simulink model "MyControl3"  (R2020b)
settings: Solver=FixedStepAuto  StartTime=0.0  StopTime=100  RelTol=1e-3
undefined symbols (not defined in the file or in its folder): ld, Ts
libraries: Solver_SF x1, simulink x1
settings Model: Creator=Namo  LastModifiedBy=Namo

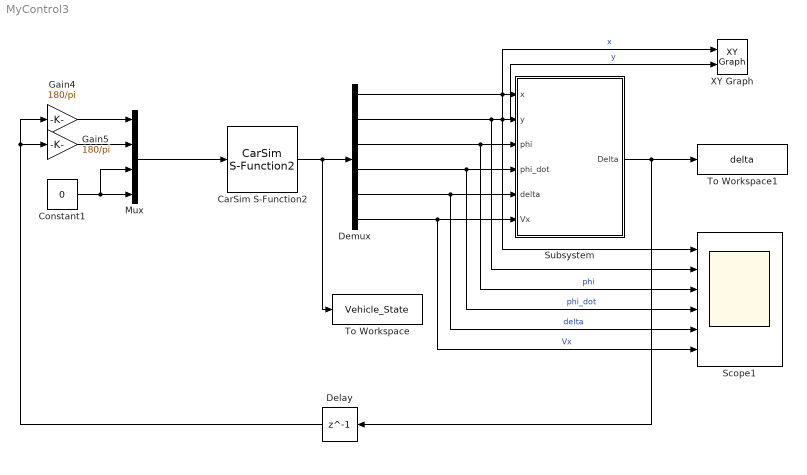
== system MyControl3 ==
  CarSim S-Function2 : Solver_SF/CarSim S-Function2  Priority=1  VehicleCode=i_i  SIMFILE=simfile.sim
      settings: AttributesFormatString=Vehicle Code: %<VehicleCode>
  Constant1 : Constant  Value=0
  Delay : Delay  DelayLength=1
  Demux : Demux  Outputs=6
  Gain4 : Gain  Gain=180/pi
  Gain5 : Gain  Gain=180/pi
  Mux : Mux
  Scope1 : Scope  NumInputPorts=6
  Subsystem : Subsystem
  To Workspace : ToWorkspace  VariableName=Vehicle_State  SampleTime=Ts
  To Workspace1 : ToWorkspace  VariableName=delta  SampleTime=-1
  XY Graph : simulink/Sinks/XY Graph  xmin=-5  xmax=200  ymin=-1  ymax=220  st=-1
  wires:
  Gain4/1 -> Mux/1
  Constant1/1 -> Mux/4, Mux/3
  CarSim S-Function2/1 -> To Workspace/1, Demux/1
  Subsystem/1(Delta) -> Delay/1, To Workspace1/1
  Mux/1 -> CarSim S-Function2/1
  Demux/6 -> Subsystem/6(Vx), Scope1/6  "Vx"
  Delay/1 -> Gain4/1, Gain5/1
  Demux/5 -> Scope1/5, Subsystem/5(delta)  "delta"
  Demux/3 -> Scope1/3, Subsystem/3(phi)  "phi"
  Gain5/1 -> Mux/2
  Demux/1 -> Scope1/1, XY Graph/1, Subsystem/1(x)  "x"
  Demux/2 -> XY Graph/2, Subsystem/2(y), Scope1/2  "y"
  Demux/4 -> Scope1/4, Subsystem/4(phi_dot)  "phi_dot"

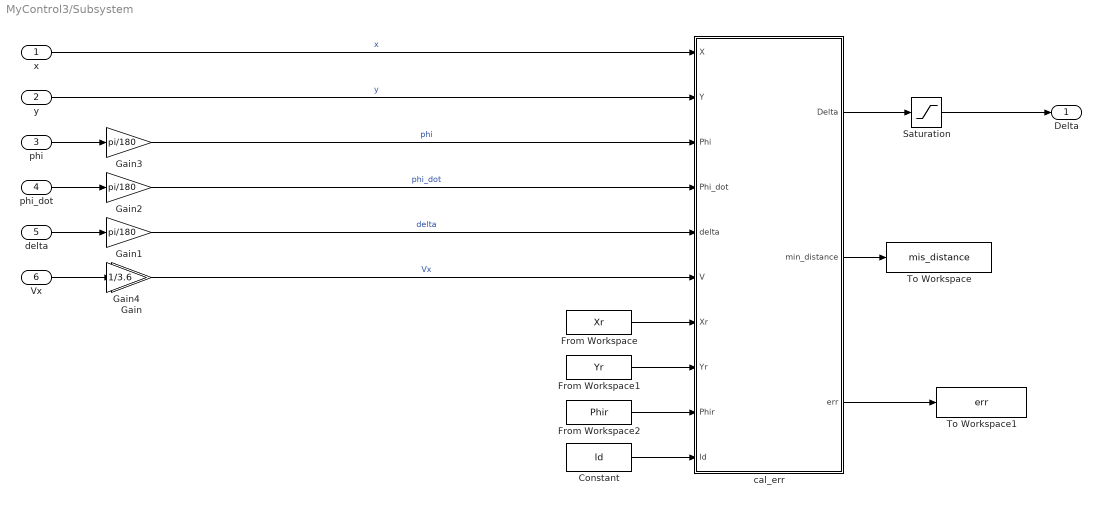
== system MyControl3/Subsystem ==
  x : Inport
  y : Inport  Port=2
  phi : Inport  Port=3
  phi_dot : Inport  Port=4
  delta : Inport  Port=5
  Vx : Inport  Port=6
  Constant : Constant  Value=ld
  From Workspace : FromWorkspace  VariableName=Xr
  From Workspace1 : FromWorkspace  VariableName=Yr
  From Workspace2 : FromWorkspace  VariableName=Phir
  Gain : Gain  Gain=1/3.6
  Gain1 : Gain  Gain=pi/180
  Gain2 : Gain  Gain=pi/180
  Gain3 : Gain  Gain=pi/180
  Gain4 : Gain  Gain=1/3.6
  Saturation : Saturate  UpperLimit=0.43  LowerLimit=-0.43
  To Workspace : ToWorkspace  VariableName=mis_distance  SampleTime=-1
  To Workspace1 : ToWorkspace  VariableName=err  SampleTime=-1
  cal_err : MATLAB Function  TreatAsAtomicUnit=on  SystemSampleTime=Ts
  Delta : Outport
  wires:
  Gain/1 -> cal_err/6(V)  "Vx"
  From Workspace1/1 -> cal_err/8(Yr)
  From Workspace/1 -> cal_err/7(Xr)
  From Workspace2/1 -> cal_err/9(Phir)
  y/1 -> cal_err/2(Y)  "y"
  Gain2/1 -> cal_err/4(Phi_dot)  "phi_dot"
  Gain1/1 -> cal_err/5(delta)  "delta"
  Gain3/1 -> cal_err/3(Phi)  "phi"
  phi/1 -> Gain3/1
  Vx/1 -> Gain/1
  phi_dot/1 -> Gain2/1
  delta/1 -> Gain1/1
  x/1 -> cal_err/1(X)  "x"
  Saturation/1 -> Delta/1
  cal_err/1(Delta) -> Saturation/1
  cal_err/2(min_distance) -> To Workspace/1
  cal_err/3(err) -> To Workspace1/1
  Constant/1 -> cal_err/10(ld)

== matlab function MyControl3/Subsystem/cal_err ==
  data: X input; Delta output; Y input; Phi input; Phi_dot input; delta input; V input; Xr input; Yr input; Phir input; min_distance output; err output; ld input
function [Delta,min_distance,err]  = cal_delta(X,Y,Phi,Phi_dot,delta,V,Xr,Yr,Phir,ld)
% 用于计算前轮偏转角的程序 预瞄控制
%   X Y Phi Phi_dot delta V 是当前车辆状态，Xr,Yr，Phir是规划轨迹点序列 Ts是采样时间 T是预设时间
tic

plot(X,Y,'.');
hold on
L = 2.7; % 车身长
Ld0 =ld  ; % 基础前视距离
kv = 0.3;
disp('Now coord:');
fprintf('X = %f,Y = %f,Phi = %f Phi_dot = %f delta = %f V = %f\n', X,Y,Phi,Phi_dot,delta,V);
%通过质心位置求得后轮中心位置
X_tran = -1.35;
Y_tran = 0;
X1 = X_tran * cos(Phi)-Y_tran*sin(Phi)+X;
Y1 = X_tran *sin(Phi) +Y_tran*cos(Phi)+Y;
X = X1;
Y = Y1;

n = length(Xr);
dist = zeros(n,1); % 寻找预瞄距离范围内最近路径点
for j = 1:n
    dist(j) = sqrt((Xr(j) -   X)^2 + (Yr(j) - Y)^2);
end
[min_distance,idx] = min(dist);

% 求最近点横向误差
d_err = [X - Xr(idx); Y - Yr(idx)];
nor = [-sin(Phir(idx));cos(Phir(idx))];
err = nor' * d_err;
fprintf('err = %f\n',err); 
fprintf('idx = %f mis_distance = %f\n',idx,min_distance);


% 从该点开始向轨迹前方搜索，找到与预瞄距离最相近的一个轨迹点
dis_sum = 0;    % 参考轨迹上几个相邻点的累计距离
% Ld = kv*V + Ld0; % Ld0 是预瞄距离的下限值
Ld = ld;
% Ld = 4;
% Ld = 25
fprintf('Ld = %f\n', Ld);
while dis_sum < Ld && idx < n
    dis_sum = dis_sum + sqrt((Xr(idx+1) - Xr(idx))^2 + (Yr(idx+1) - Yr(idx))^2);
    idx = idx+1;
end
idx_target = idx;
fprintf('idx_target = %f\n', idx_target); 

% % % 
% X_tran = -1.35;
% Y_tran = 0;
% X1 = X_tran * cos(Phi)-Y_tran*sin(Phi)+X;
% Y1 = X_tran *sin(Phi) +Y_tran*cos(Phi)+Y;
% X = X1;
% Y = Y1;


%% 获得控制量：前轮转角
alpha = atan2(Yr(idx_target) - Y, Xr(idx_target)-X) - Phi;
Delta = atan2(2*L*sin(alpha),Ld);  

toc
end
